simulink model "problem2_"  (R2020b)
settings: Solver=FixedStepDiscrete  StartTime=0.0  StopTime=150  FixedStep=.1  RelTol=1e-3  EnableMultiTasking=on
undefined symbols (not defined in the file): DiscIntNeverNeededParam
libraries: simulink x1
settings Model: Creator=The MathWorks, Inc.  LastModifiedBy=Hp
settings DataIOCC: LimitDataPoints=on  SaveFormat=Array  ReturnWorkspaceOutputs=off
settings OptimizationCC: ExpressionDepthLimit=2147483647  InitFltsAndDblsToZero=on  EfficientMapNaN2IntZero=off  LifeSpan=inf
settings DebuggingCC: SaveWithParameterizedLinksMsg=none  UnderspecifiedInitializationDetection=Classic  MergeDetectMultiDrivingBlocksExec=none  SignalResolutionControl=TryResolveAllWithWarning  SolverPrmCheckMsg=warning  MultiTaskDSMMsg=warning  MultiTaskCondExecSysMsg=none  FcnCallInpInsideContextMsg=warning  StateNameClashWarn=warning  SFUnexpectedBacktrackingDiag=warning  SFNoUnconditionalDefaultTransitionDiag=warning  SFExecutionAtInitializationDiag=none  ArithmeticOperatorsInVariantConditions=warning
settings HardwareCC: ProdBitPerPointer=32  ProdBitPerSizeT=32  ProdBitPerPtrDiffT=32  ProdLargestAtomicFloat=None  ProdIntDivRoundTo=Undefined  ProdEndianess=Unspecified  ProdWordSize=32  ProdHWDeviceType=32-bit Generic
settings ModelReferenceCC: PropagateSignalLabelsOutOfModel=off
settings SFSimCC: SimUseLocalCustomCode=off  SimParseCustomCode=off  CustomCodeUndefinedFunction=UseInterfaceOnly
settings RTWCC: RTWUseLocalCustomCode=off
settings CodeAppCC: StateflowObjectComments=on
settings GRTTargetCC: TargetFcnLib=ansi_tfl_tmw.mat  TargetLangStandard=C89/C90 (ANSI)  CombineOutputUpdateFcns=off  GRTInterface=on
settings ConfigComp: CovMetricSettings=dw  CovSaveCumulativeToWorkspaceVar=on  CovSaveSingleToWorkspaceVar=on  CovExternalEMLEnable=off  CovSFcnEnable=off

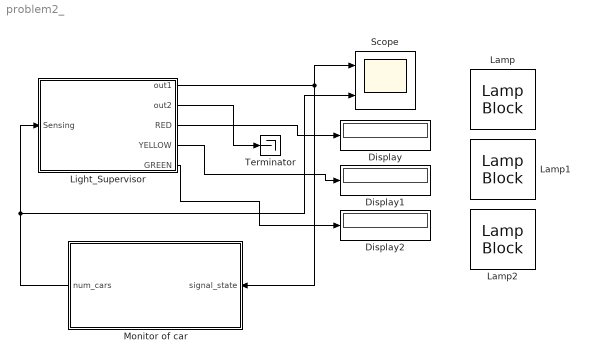
== system problem2_ ==
  Display : Display
  Display1 : Display
  Display2 : Display
  Lamp : LampBlock
  Lamp1 : LampBlock
  Lamp2 : LampBlock
  Light_Supervisor : Stateflow chart  TreatAsAtomicUnit=on
  Monitor of car : Subsystem
  Scope : Scope  NumInputPorts=2
  Terminator : Terminator
  wires:
  Light_Supervisor/2(out2) -> Terminator/1
  Light_Supervisor/1(out1) -> Monitor of car/1(signal_state), Scope/1
  Monitor of car/1(num_cars) -> Light_Supervisor/1(Sensing), Scope/2
  Light_Supervisor/3(RED) -> Display/1
  Light_Supervisor/4(YELLOW) -> Display1/1
  Light_Supervisor/5(GREEN) -> Display2/1

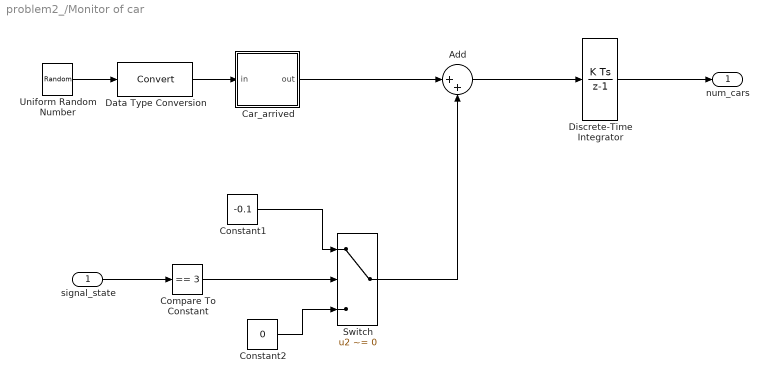
== system problem2_/Monitor of car ==
  signal_state : Inport
  Add : Sum  Inputs=|++
  Car_arrived : Stateflow chart  TreatAsAtomicUnit=on
  Compare To Constant : simulink/Logic and Bit Operations/Compare To Constant  relop===  const=3  OutDataTypeStr=boolean  ZeroCross=off
  Constant1 : Constant  Value=-0.1
  Constant2 : Constant  Value=0
  Data Type Conversion : DataTypeConversion
  Discrete-Time Integrator : DiscreteIntegrator  SampleTime=-1  LimitOutput=on  LowerSaturationLimit=0  ICPrevOutput=DiscIntNeverNeededParam  ICPrevScaledInput=DiscIntNeverNeededParam
  Switch : Switch  Criteria=u2 ~= 0
  Uniform Random Number : UniformRandomNumber  Minimum=0  Maximum=100  Seed=177836  SampleTime=0
  num_cars : Outport  VectorParamsAs1DForOutWhenUnconnected=off
  wires:
  Constant1/1 -> Switch/1
  Constant2/1 -> Switch/3
  Discrete-Time Integrator/1 -> num_cars/1
  signal_state/1 -> Compare To Constant/1
  Compare To Constant/1 -> Switch/2
  Switch/1 -> Add/2
  Add/1 -> Discrete-Time Integrator/1
  Car_arrived/1(out) -> Add/1
  Data Type Conversion/1 -> Car_arrived/1(in)
  Uniform Random Number/1 -> Data Type Conversion/1

== stateflow chart problem2_/Light_Supervisor ==
  settings: stateMachineType=MOORE_MACHINE  executeAtInitialization=1  initializeOutput=1
  state Stop
    RED=1;
    GREEN=0;
    YELLOW=0;
    out1 = RED;
    out2 = GREEN;
  state StopToGo
    RED=1;
    GREEN=0;
    YELLOW=0;
    out1 = RED;
    out2 = YELLOW;
  state StopForTraffic
    RED=1;
    GREEN=0;
    YELLOW=0;
    out1 = RED;
    out2 = GREEN;
  state GoToStop
    out1 = YELLOW;
    out2 = RED;
    RED=0;
    GREEN=0;
    YELLOW=1;
  state Go
    out1 = GREEN;
    out2 = RED;
    RED=0;
    GREEN=1;
    YELLOW=0;
  (default) -> Stop
  StopForTraffic -> StopToGo : [Sensing]
  Stop -> StopForTraffic : after(30,tick)
  GoToStop -> Stop : after (4,tick)
  StopToGo -> Go : after(4,tick)
  Go -> GoToStop : after(20,tick)
  data: Sensing input double; out1 output double; out2 output double; RED output uint8 =1; YELLOW output double =2; GREEN output double =3

== stateflow chart problem2_/Monitor of car/Car_arrived ==
  (default) -> (junction 2) : {out = in > 98;}
  data: in input int8; out output double
